simulink subsystem "ClampVal"  (R2022a)
settings: Solver=VariableStepAuto  StartTime=0.0  StopTime=10.0  RelTol=1e-3
settings Model: Creator=bkfre  LastModifiedBy=bkfre

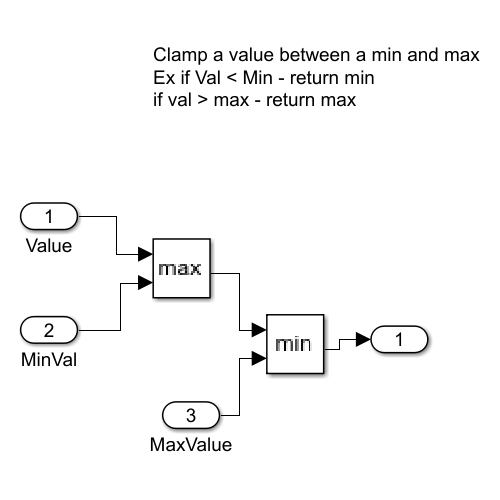
[thumbnail: Simulink's stored preview of the top-level diagram]
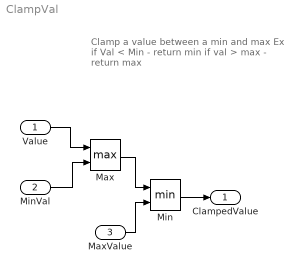
== system ClampVal ==
  note: Clamp a value between a min and max
      | Ex if Val < Min - return min
      | if val > max - return max
  Value : Inport
  MinVal : Inport  Port=2
  MaxValue : Inport  Port=3
  Max : MinMax  Function=max  Inputs=2
  Min : MinMax  Inputs=2
  ClampedValue : Outport
  wires:
  Min/1 -> ClampedValue/1
  MaxValue/1 -> Min/2
  Value/1 -> Max/1
  MinVal/1 -> Max/2
  Max/1 -> Min/1
